simulink model "TRAMI_STEP_AT_vehicle_ver01_Jmaab_R2018b"  (R2018b)
settings: Solver=ode8  StartTime=0  StopTime=end_time  FixedStep=sampling_time  RelTol=1e-3
PreLoadFcn:
  | %init_setting;
values from neighbouring files (symbols this model uses):
  sampling_time = 0.0025    [METI_TRAMI_Thermal_ver01_Jmaab_PreLoad.m]
undefined symbols (not defined in the file or in its folder): ACC_D_Gain, ACC_I_Gain, ACC_P_Gain, ALT_CNT_ALT_OFF_RPM_HYS_rpm, ALT_CNT_ALT_ON_RPM_HYS_rpm, ALT_CNT_Alter_V_BASE_V, ALT_CNT_Alter_V_Kaisei_V, ALT_CNT_flag_disable_kaisei, ALT_CNT_V_Battely_Kudo_V, ALT_PNT_ALT_GDCurrent_A, ALT_PNT_ALT_GDVolt_V, ALT_PNT_Alter_limit_Current_V_table, ALT_PNT_Alter_limit_Current_V_table_x_rpm, ALT_PNT_Alter_trq_Nm_map, ALT_PNT_Alter_trq_Nm_map_x_rpm, ALT_PNT_Alter_trq_Nm_map_y_Current_A, ALT_PNT_Alter_trq_Nm_map_z_Volt_tgt_V, ALT_PNT_eta_pulley_alt, ALT_PNT_Gain_Alt_v_del, ALT_PNT_ratio_pulley_alt, ALT_PNT_Tau_Alternator_V_tgt_s, ALT_PNT_trq_alter_output_LL_Nm, BK_PNT_Pow_UL, BK_PNT_Tau_brake, Brk_LL, Brk_PGain, Brk_UL, BT_PNT_Lo_Capa_lo_batt_F, BT_PNT_Lo_ocv_SOC_lo_batt_OCV_V_table, BT_PNT_Lo_ocv_SOC_lo_batt_OCV_V_table_x_SOC, BT_PNT_Lo_R_lo_batt_ohm, BT_PNT_Lo_SOC_MAX_lo_batt, BT_PNT_Lo_SOC_MIN_lo_batt, BT_PNT_Lo_SOC_START_lo_batt, BT_PNT_Lo_V_start_ocv, DF_PNT_DF_gear, Driver_Brake_Const1, Driver_Brake_Const3, Driver_Brake_Switch_Const2, Driver_Brk_sh, drivmode_ACC, drivmode_CONST, drivmode_GensokuKaisei, drivmode_GensokuRikko, drivmode_STOP, EL_PNT_R_bodyelec_lo_ohm, ENG_CNT_Accel_LL, ENG_CNT_Accel_UL, ENG_CNT_brak_idlestop, ENG_CNT_flag_idle_stop_exe, ENG_CNT_gain_p_per_isc, ENG_CNT_IdleSpeed_Const, ENG_CNT_omg_eng_fuelcut_rpm, ENG_CNT_per_isc_max, ENG_CNT_per_isc_min, ENG_CNT_per_throttle_fuelcut, ENG_CNT_per_throttle_isc_fb, ENG_CNT_Starter_timer_Const_s, ENG_CNT_Throttle_LL, ENG_CNT_Throttle_UL ... (+31)
libraries: METI_Lib_vehicle_model x18, simulink x4, AZAPA_Lib_vehicle_model x1
(part 2 of 3)

== system TRAMI_STEP_AT_vehicle_ver01_Jmaab_R2018b/Vehicle/CNT/TM_CNT ==
  sensor_VL_PNT_BUS : Inport
  sensor_TM_PNT_BUS : Inport  Port=2
  Bus Creator : BusCreator  Inputs=2
  Bus Creator2 : BusCreator  Inputs=12
  Bus Selector1 : BusSelector  OutputSignals=open_accel_per,trq_BK_PNT_Nm,IdleSpeed_Target
  Bus Selector11 : BusSelector  OutputSignals=w_TM_PNT_GearBox_in_radps,w_TM_PNT_GearBox_out_radps,wDiff,T_oil_K,w_TM_PNT_out_radps,trq_FW_PNT_in_unLim_Nm,trq_FW_PNT_in_Nm
  Bus Selector3 : BusSelector  OutputSignals=v_VL_PNT_kmph
  Constant : Constant  Value=500
  Constant1 : Constant  Value=0
  Gain : Gain  Gain=2*pi/60
  Gain1 : Gain  Gain=-1
  Step : Step  Time=5.57  SampleTime=0
  T_PT_TH_K : Subsystem
  Terminator1 : Terminator
  Terminator2 : Terminator
  plant_Connection : Subsystem
  TM_CNT_out : Outport
  tag scope: TM_CNT_CAN_Tx=scoped
  wires:
  Bus Creator/1 -> [TM_CNT_CAN_Tx]  "TM_CNT_CAN_Tx"
  [TM_CNT_CAN_Rx] -> Bus Selector1/1
  Bus Selector1/1 -> plant_Connection/6(accel_position_per)  "<open_accel_per>"
  sensor_VL_PNT_BUS/1 -> Bus Selector3/1
  Bus Selector11/4 -> plant_Connection/4(t_trans_fluid_k)  "<T_oil_K>"
  Bus Selector11/7 -> plant_Connection/13(tau_engine)  "<trq_FW_PNT_in_Nm>"
  Bus Selector11/6 -> plant_Connection/12(tau_engine_target)  "<trq_FW_PNT_in_unLim_Nm>"
  plant_Connection/9(tq_engine_min_req) -> Bus Creator2/9
  plant_Connection/13(flag_lock_up) -> Bus Creator/1, Bus Creator2/11
  plant_Connection/12(gear_ratio) -> Bus Creator/2, Bus Creator2/10
  plant_Connection/7(q_cooler_engine_water) -> Bus Creator2/7
  plant_Connection/6(q_cooler_trans_fluid) -> Bus Creator2/6
  plant_Connection/1(tq_clutch_cap) -> Bus Creator2/1
  plant_Connection/8(tq_engine_max_req) -> Bus Creator2/8
  T_PT_TH_K/1(Out1) -> plant_Connection/5(t_engine_water_k)
  Bus Creator2/1 -> TM_CNT_out/1  "TM_CNT_out"
  Constant/1 -> plant_Connection/15(tau_engine_max_pos)
  plant_Connection/5(i_eop) -> Bus Creator2/5
  plant_Connection/14(lock_up_cap) -> Bus Creator2/12
  Bus Selector11/2 -> plant_Connection/2(w_gearbox_output_radps)  "<w_TM_PNT_GearBox_out_radps>"
  Gain/1 -> plant_Connection/11(w_engine_idle_radps)
  Step/1 -> plant_Connection/7(trans_shifer_position)
  Constant1/1 -> plant_Connection/14(tau_engine_min_pos)
  plant_Connection/3(p_line) -> Bus Creator2/3
  plant_Connection/11(tq_trans_input) -> Terminator2/1
  Bus Selector11/1 -> plant_Connection/1(w_gearbox_input_radps)  "<w_TM_PNT_GearBox_in_radps>"
  plant_Connection/4(i_actuator) -> Bus Creator2/4
  Gain1/1 -> plant_Connection/9(tau_brake)
  sensor_TM_PNT_BUS/1 -> Bus Selector11/1
  plant_Connection/10(r_engine_target) -> Terminator1/1
  Bus Selector11/3 -> plant_Connection/3(w_synchoro_dif_radps)  "<wDiff>"
  plant_Connection/2(f_synchro_n) -> Bus Creator2/2
  Bus Selector11/5 -> plant_Connection/10(w_engine_radps)  "<w_TM_PNT_out_radps>"
  Bus Selector3/1 -> plant_Connection/8(v_vehicle_mps)  "<v_VL_PNT_kmph>"
  Bus Selector1/3 -> Gain/1  "<IdleSpeed_Target>"
  Bus Selector1/2 -> Gain1/1  "<trq_BK_PNT_Nm>"

== system TRAMI_STEP_AT_vehicle_ver01_Jmaab_R2018b/Vehicle/ENG_PNT/ENG_Plant ==
  note: 軸トルクマップ
  note: 燃料消費率マップ
  open_throttle_per : Inport
  flag_fuelcut : Inport  Port=2
  flag_IdleStop : Inport  Port=3
  timing_ignition : Inport  Port=4
  w_ENG_PNT_radps : Inport  Port=5
  Cal_FuelComsunption : Subsystem
  Cal_trq_ENG_jiku : Subsystem
  Gain : Gain  Gain=radpsec2rpm
  Integrator : Integrator
  Model Info : simulink/Model-Wide Utilities/Model Info  Frame=on  DisplayStringWithTags=【注記】 ・エンジンモデルはトルク出力動作させる側が正  HorizontalTextAlignment=Left  LeftAlignmentValue=0.02
  P_cal : METI_Lib_vehicle_model/P_cal  Type_energy=回転運動  Type_output_energy=出力  Power_name=Po_  t_Workspace_Name=ENG_PNT_MECK  P_VariableName=Po_ENG_PNT_MECK  Across_VariableName=w_ENG_PNT_MECK  Throgh_VariableName=tq_ENG_PNT_MECK
  Terminator1 : Terminator
  n_eng_rpm : Outport
  trq_ENG_PNT_Nm : Outport  Port=2
  tag scope: tScope_ENG_speed_rpm=global, tScope_ENG_torq=global, tScope_Fuel=global, tScope_Fuelraio=global
  wires:
  w_ENG_PNT_radps/1 -> Cal_trq_ENG_jiku/5(w_ENG_PNT_radps), P_cal/1, Gain/1, Cal_FuelComsunption/1(w_ENG_PNT_radps)
  Cal_FuelComsunption/1(FuelComsunption) -> [tScope_Fuelraio], Integrator/1
  flag_fuelcut/1 -> Cal_trq_ENG_jiku/2(flag_fuelcut), Cal_FuelComsunption/3(flag_fuelcut)
  flag_IdleStop/1 -> Cal_FuelComsunption/4(flag_IdleStop), Cal_trq_ENG_jiku/3(flag_IdleStop)
  P_cal/1 -> Terminator1/1
  open_throttle_per/1 -> Cal_trq_ENG_jiku/1(open_throttle_per)
  timing_ignition/1 -> Cal_FuelComsunption/5(timing_ignition), Cal_trq_ENG_jiku/4(timing_ignition)
  Integrator/1 -> [tScope_Fuel]
  Gain/1 -> [tScope_ENG_speed_rpm], n_eng_rpm/1  "n_eng_rpm"
  Cal_trq_ENG_jiku/1(trq_ENG_PNT_Nm) -> Cal_FuelComsunption/2(trq_ENG), [tScope_ENG_torq], trq_ENG_PNT_Nm/1, P_cal/2

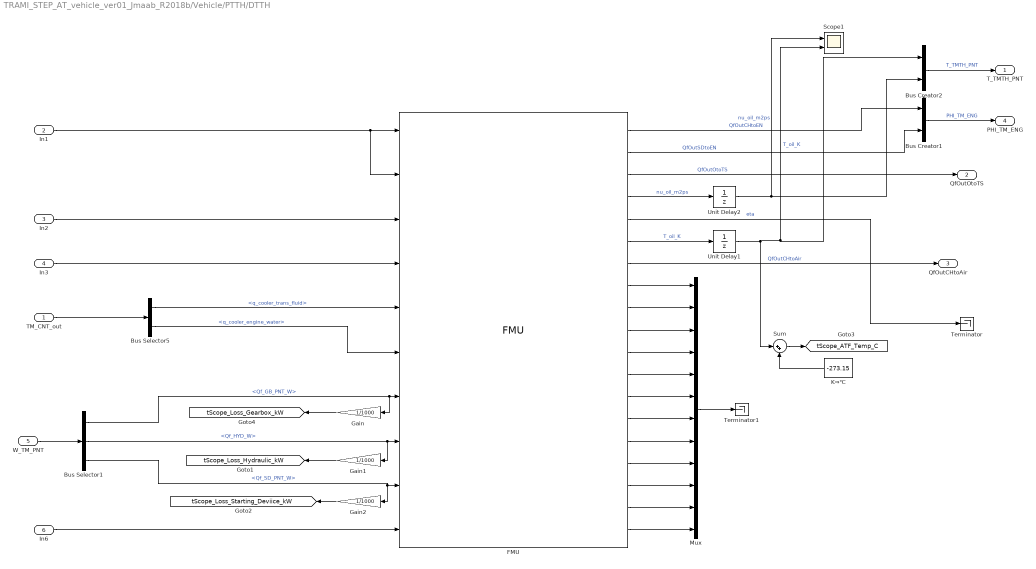
== system TRAMI_STEP_AT_vehicle_ver01_Jmaab_R2018b/Vehicle/PTTH/DTTH ==
  TM_CNT_out : Inport
  In1 : Inport  Port=2
  In2 : Inport  Port=3
  In3 : Inport  Port=4
  W_TM_PNT : Inport  Port=5
  In6 : Inport  Port=6
  Bus Creator1 : BusCreator  Inputs=2
  Bus Creator2 : BusCreator  Inputs=2
  Bus Selector1 : BusSelector  OutputSignals=Qf_GB_PNT_W,Qf_HYD_W,Qf_SD_PNT_W
  Bus Selector5 : BusSelector  OutputSignals=q_cooler_trans_fluid,q_cooler_engine_water
  FMU : FMU  FMUName=ThermalModelAll_CS.fmu  FMUDebugLogging=on  FMUMode=CoSimulation  c1=5000  T0=300  R1=100  T1=300  R2=0.10  R3=100  R4=100  R5=0.006  table1_1_1__1_1_=0.  table1_1_2__1_2_=0.022  table1_2_1__2_1_=10.  table1_2_2__2_2_=0.021  table1_3_1__3_1_=20.  table1_3_2__3_2_=0.021  table1_4_1__4_1_=30.  table1_4_2__4_2_=0.020  table1_5_1__5_1_=40.  table1_5_2__5_2_=0.019  table1_6_1__6_1_=50.  table1_6_2__6_2_=0.018  table1_7_1__7_1_=60.  table1_7_2__7_2_=0.017  table1_8_1__8_1_=70.  table1_8_2__8_2_=0.016  table1_9_1__9_1_=80.  table1_9_2__9_2_=0.015  table1_10_1__10_1_=90.  table1_10_2__10_2_=0.014  table1_11_1__11_1_=100.  table1_11_2__11_2_=0.013  table1_12_1__12_1_=110.  table1_12_2__12_2_=0.012  table1_13_1__13_1_=120.  table1_13_2__13_2_=0.012  table1_14_1__14_1_=130.  table1_14_2__14_2_=0.011  table1_15_1__15_1_=140.  table1_15_2__15_2_=0.011  table1_16_1__16_1_=150.  table1_16_2__16_2_=0.010  table1_17_1__17_1_=160.  table1_17_2__17_2_=0.010  c3=15000  T2=300  fileName1=./DATA/thResistanceOilColler1.txt  tableName1=thResistanceOilColler1  T3=300  c4=10000  R6=0.0007  R7=0.05  Nutable1_1_1__1_1_=-30.  Nutable1_1_2__1_2_=70  Nutable1_2_1__2_1_=0.  Nutable1_2_2__2_2_=70  Nutable1_3_1__3_1_=20.  Nutable1_3_2__3_2_=70  Nutable1_4_1__4_1_=40.  Nutable1_4_2__4_2_=40  Nutable1_5_1__5_1_=60.  Nutable1_5_2__5_2_=23  Nutable1_6_1__6_1_=80.  Nutable1_6_2__6_2_=13  Nutable1_7_1__7_1_=100.  Nutable1_7_2__7_2_=7.5  Nutable1_8_1__8_1_=120.  Nutable1_8_2__8_2_=7.5  EtaTable1_1_1__1_1_=-30.  EtaTable1_1_2__1_2_=70  EtaTable1_2_1__2_1_=0.  EtaTable1_2_2__2_2_=70  EtaTable1_3_1__3_1_=20.  EtaTable1_3_2__3_2_=70  EtaTable1_4_1__4_1_=40.  EtaTable1_4_2__4_2_=40  EtaTable1_5_1__5_1_=60.  EtaTable1_5_2__5_2_=23  EtaTable1_6_1__6_1_=80.  EtaTable1_6_2__6_2_=13  EtaTable1_7_1__7_1_=100.  EtaTable1_7_2__7_2_=7.5  EtaTable1_8_1__8_1_=120.  EtaTable1_8_2__8_2_=7.5  kDammy=1.  c2=30000  settings_dtMin=1e-08  settings_dtMax=0.01  settings_absTol=1e-05  settings_relTol=1e-05  settings_iMode=int32(1)  settings_maxOrder=int32(5)  mask(ThermalModelAll [Co-Simulation, v2.0]){}
      mask Display:
      | disp('ThermalModelAll');
      | port_label('output',1,'QfOutCHtoEN');
      | port_label('output',2,'QfOutSDtoEN');
      | port_label('output',3,'QfOutOCtoTS');
      | port_label('output',4,'nuOil');
      | port_label('output',5,'etaOil');
      | port_label('output',6,'ToutOil');
      | port_label('output',7,'QfOutCHtoAir');
      | port_label('output',8,'ToutOiltoOC');
      | port_label('output',9,'QfOutOCtoOil');
      | port_label('output',10,'ToutSDtoOil');
      | port_label('output',11,'QfOutOiltoSD');
      | port_label('output',12,'ToutSDtoCH');
      | port_label('output',13,'QfOutCHtoSD');
      | port_label('output',14,'ToutOiltoCH');
      | port_label('output',15,'QfoutCHtoOil');
      | port_label('output',16,'QfOiltoGear');
      | port_label('output',17,'ToutGeartoOil');
      | port_label('output',18,'ToutGeartoCH');
      | port_label('output',19,'QfOutCHtoGear');
      | port_label('input',1,'TinENtoCH');
      | port_label('input',2,'TinENtoSD');
      | port_label('input',3,'TinTStoOC');
      | port_label('input',4,'TinAirtoCH');
      | port_label('input',5,'VIdot1OilCooler');
      | port_label('input',6,'VIdot2OilCooler');
      | port_label('input',7,'QfGear');
      | port_label('input',8,'QfOil');
      | port_label('input',9,'QfStartDevice');
      | port_label('input',10,'vCaseHousing');
  Gain : Gain  Gain=1/1000
  Gain1 : Gain  Gain=1/1000
  Gain2 : Gain  Gain=1/1000
  K⇒℃ : Constant  Value=-273.15
  Mux : Mux  Inputs=12
  Scope1 : Scope  NumInputPorts=2
  Sum : Sum  Inputs=|++
  Terminator : Terminator
  Terminator1 : Terminator
  Unit Delay1 : UnitDelay  InitialCondition=8e-5  SampleTime=-1
  Unit Delay2 : UnitDelay  InitialCondition=8e-5  SampleTime=-1
  T_TMTH_PNT : Outport
  QfOutOtoTS : Outport  Port=2
  QfOutCHtoAir : Outport  Port=3
  PHI_TM_ENG : Outport  Port=4
  tag scope: tScope_ATF_Temp_C=global, tScope_Loss_Gearbox_kW=global, tScope_Loss_Hydraulic_kW=global, tScope_Loss_Starting_Deviice_kW=global
  wires:
  FMU/14 -> Mux/7
  Unit Delay2/1 -> Scope1/1, Bus Creator2/2  "nu_oil_m2ps"
  Bus Selector1/1 -> Gain/1, FMU/7  "<Qf_GB_PNT_W>"
  K⇒℃/1 -> Sum/2
  Gain1/1 -> [tScope_Loss_Hydraulic_kW]
  Gain/1 -> [tScope_Loss_Gearbox_kW]
  Unit Delay1/1 -> Bus Creator2/1, Scope1/2, Sum/1  "T_oil_K"
  W_TM_PNT/1 -> Bus Selector1/1
  Gain2/1 -> [tScope_Loss_Starting_Deviice_kW]
  Sum/1 -> [tScope_ATF_Temp_C]
  FMU/18 -> Mux/11
  FMU/16 -> Mux/9
  TM_CNT_out/1 -> Bus Selector5/1
  In1/1 -> FMU/2, FMU/1
  FMU/2 -> Bus Creator1/2  "QfOutSDtoEN"
  FMU/12 -> Mux/5
  FMU/4 -> Unit Delay2/1  "nu_oil_m2ps"
  FMU/17 -> Mux/10
  FMU/8 -> Mux/1
  FMU/19 -> Mux/12
  Bus Selector1/2 -> Gain1/1, FMU/8  "<Qf_HYD_W>"
  FMU/11 -> Mux/4
  FMU/10 -> Mux/3
  FMU/9 -> Mux/2
  Bus Selector1/3 -> Gain2/1, FMU/9  "<Qf_SD_PNT_W>"
  FMU/15 -> Mux/8
  Mux/1 -> Terminator1/1
  FMU/13 -> Mux/6
  FMU/6 -> Unit Delay1/1  "T_oil_K"
  FMU/5 -> Terminator/1  "eta"
  Bus Selector5/2 -> FMU/6  "<q_cooler_engine_water>"
  In6/1 -> FMU/10
  Bus Selector5/1 -> FMU/5  "<q_cooler_trans_fluid>"
  FMU/7 -> QfOutCHtoAir/1  "QfOutCHtoAir"
  FMU/3 -> QfOutOtoTS/1  "QfOutOtoTS"
  In2/1 -> FMU/3
  In3/1 -> FMU/4
  FMU/1 -> Bus Creator1/1  "QfOutCHtoEN"
  Bus Creator2/1 -> T_TMTH_PNT/1  "T_TMTH_PNT"
  Bus Creator1/1 -> PHI_TM_ENG/1  "PHI_TM_ENG"

== system TRAMI_STEP_AT_vehicle_ver01_Jmaab_R2018b/Vehicle/PTTH/ENGTH ==
  PHI_TM_ENG : Inport
  Bus Selector : BusSelector  OutputSignals=QfOutCHtoEN,QfOutSDtoEN
  From Workspace1 : FromWorkspace  VariableName=T_ENG_K  SampleTime=0  OutputAfterFinalValue=Holding final value
  Sum : Sum  Inputs=|++
  Terminator : Terminator
  Terminator1 : Terminator
  ℃⇒K : Constant  Value=273.15
  T_ENG_K : Outport
      settings: AttributesFormatString=|
      | %<Tag>
      | Priority=<%<Priority>>
  wires:
  Bus Selector/2 -> Terminator/1  "<QfOutSDtoEN>"
  From Workspace1/1 -> Sum/1
  ℃⇒K/1 -> Sum/2
  Sum/1 -> T_ENG_K/1  "T_ENG_K"
  PHI_TM_ENG/1 -> Bus Selector/1
  Bus Selector/1 -> Terminator1/1  "<QfOutCHtoEN>"

== system TRAMI_STEP_AT_vehicle_ver01_Jmaab_R2018b/Vehicle/PTTH/PT_TH ==
  Qf_cooler_PT_TH_W : Inport
      settings: AttributesFormatString=|
      | %<Tag>
      | Priority=<%<Priority>>
  From Workspace1 : FromWorkspace  VariableName=T_PT_TH_K  SampleTime=0  OutputAfterFinalValue=Holding final value
  Sum : Sum  Inputs=|++
  Terminator : Terminator
  ℃⇒K : Constant  Value=273.15
  T_PT_TH_K : Outport
      settings: AttributesFormatString=|
      | %<Tag>
      | Priority=<%<Priority>>
  wires:
  Qf_cooler_PT_TH_W/1 -> Terminator/1
  ℃⇒K/1 -> Sum/2
  From Workspace1/1 -> Sum/1
  Sum/1 -> T_PT_TH_K/1  "T_PT_TH_K"

== system TRAMI_STEP_AT_vehicle_ver01_Jmaab_R2018b/Vehicle/PTTH/air ==
  Qf_case_air_W : Inport
      settings: AttributesFormatString=|
      | %<Tag>
      | Priority=<%<Priority>>
  From Workspace1 : FromWorkspace  VariableName=T_air_K  SampleTime=0  OutputAfterFinalValue=Holding final value
  Sum : Sum  Inputs=|++
  Terminator : Terminator
  ℃⇒K : Constant  Value=273.15
  T_air_K : Outport
      settings: AttributesFormatString=|
      | %<Tag>
      | Priority=<%<Priority>>
  wires:
  Qf_case_air_W/1 -> Terminator/1
  From Workspace1/1 -> Sum/1
  ℃⇒K/1 -> Sum/2
  Sum/1 -> T_air_K/1  "T_air_K"

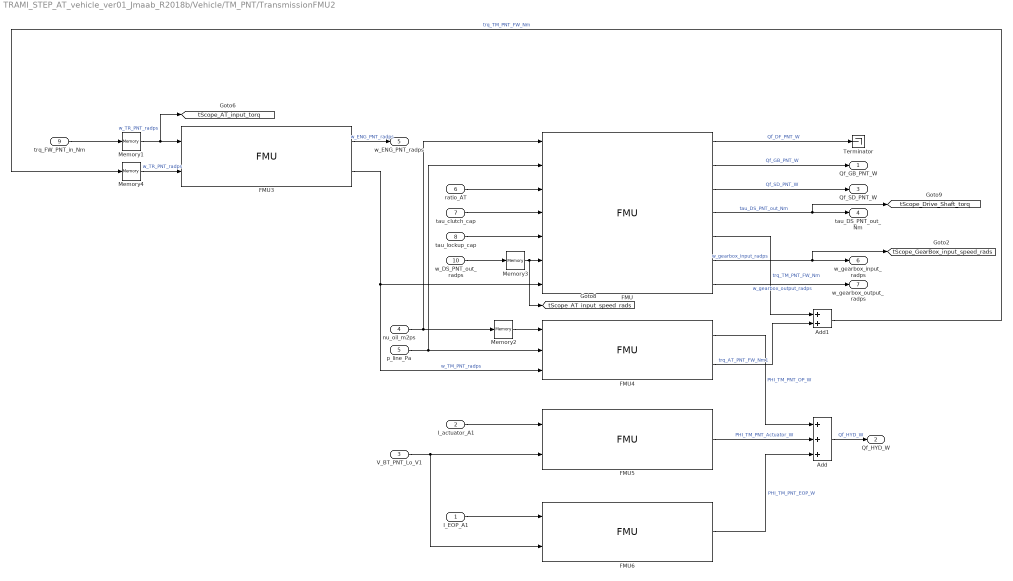
== system TRAMI_STEP_AT_vehicle_ver01_Jmaab_R2018b/Vehicle/TM_PNT/TransmissionFMU2 ==
  I_EOP_A1 : Inport
  I_actuator_A1 : Inport  Port=2
  V_BT_PNT_Lo_V1 : Inport  Port=3
  nu_oil_m2ps : Inport  Port=4
  p_line_Pa : Inport  Port=5
  ratio_AT : Inport  Port=6
  tau_clutch_cap : Inport  Port=7
  tau_lockup_cap : Inport  Port=8
  trq_FW_PNT_in_Nm : Inport  Port=9
  w_DS_PNT_out_radps : Inport  Port=10
  Add : Sum  Inputs=+++
  Add1 : Sum
  FMU : FMU  FMUName=AtDsFmu.fmu  FMUMode=CoSimulation  minsamplestep=2.50000000000000000e-02  binfilename=DISABLED  mask(AtDsFmu [Co-Simulation, v2.0]){}
      mask Display:
      | disp('AtDsFmu');
      | port_label('output',1,'Qf_DF_PNT_W');
      | port_label('output',2,'Qf_GB_PNT_W');
      | port_label('output',3,'Qf_SD_PNT_W');
      | port_label('output',4,'tau_DS_PNT_out_Nm');
      | port_label('output',5,'trq_TM_PNT_FW_Nm');
      | port_label('output',6,'w_gearbox_input_radps');
      | port_label('output',7,'w_gearbox_output_radps');
      | port_label('input',1,'nu_oil_m2ps');
      | port_label('input',2,'p_line_Pa');
      | port_label('input',3,'ratio_AT');
      | port_label('input',4,'tau_clutch_cap');
      | port_label('input',5,'tau_lockup_cap');
      | port_label('input',6,'w_DS_PNT_out_radps');
      | port_label('input',7,'w_TM_PNT_FW_radps');
  FMU3 : FMU  FMUName=Flywheel.fmu  FMUMode=CoSimulation  Iwh=4.00000000000000000e-01  minsamplestep=2.50000000000000000e-02  binfilename=DISABLED  mask(Flywheel [Co-Simulation, v2.0]){}
      mask Display:
      | disp('Flywheel');
      | port_label('output',1,'w_ENG_PNT_radps');
      | port_label('output',2,'w_TM_PNT_FW_radps');
      | port_label('input',1,'trq_ENG_PNT_in_Nm');
      | port_label('input',2,'trq_TM_PNT_FW_Nm');
  FMU4 : FMU  FMUName=OilPump.fmu  FMUMode=CoSimulation  Oil_Viscosity_Breakpoint_2=1.02000000000000000e-05  Oil_Viscosity_Breakpoint_3=1.69000000000000000e-05  Oil_Viscosity_Breakpoint_4=3.12000000000000000e-05  minsamplestep=2.50000000000000000e-02  binfilename=DISABLED  mask(OilPump [Co-Simulation, v2.0]){}
      mask Display:
      | disp('OilPump');
      | port_label('output',1,'PHI_TM_PNT_OP_W');
      | port_label('output',2,'trq_AT_PNT_Nm1');
      | port_label('input',1,'nu_oil_m2ps');
      | port_label('input',2,'p_Line_Pa');
      | port_label('input',3,'w_AT_PNT_radps1');
  FMU5 : FMU  FMUName=ActuatorELoss.fmu  FMUMode=CoSimulation  minsamplestep=2.50000000000000000e-02  binfilename=DISABLED  mask(ActuatorELoss [Co-Simulation, v2.0]){}
      mask Display:
      | disp('ActuatorELoss');
      | port_label('output',1,'PHI_TM_PNT_Actuator_W');
      | port_label('input',1,'I_actuator_A');
      | port_label('input',2,'V_BT_PNT_Lo_V');
  FMU6 : FMU  FMUName=EOPELoss.fmu  FMUMode=CoSimulation  minsamplestep=2.50000000000000000e-02  binfilename=DISABLED  mask(EOPELoss [Co-Simulation, v2.0]){}
      mask Display:
      | disp('EOPELoss');
      | port_label('output',1,'PHI_TM_PNT_EOP_W');
      | port_label('input',1,'I_EOP_A');
      | port_label('input',2,'V_BT_PNT_Lo_V');
  Memory{1..4} (4 alike) : Memory
  Terminator : Terminator
  Qf_GB_PNT_W : Outport
  Qf_HYD_W : Outport  Port=2
  Qf_SD_PNT_W : Outport  Port=3
  tau_DS_PNT_out_Nm : Outport  Port=4
  w_ENG_PNT_radps : Outport  Port=5
  w_gearbox_input_radps : Outport  Port=6
  w_gearbox_output_radps : Outport  Port=7
  tag scope: tScope_AT_input_speed_rads=global, tScope_AT_input_torq=global, tScope_Drive_Shaft_torq=global, tScope_GearBox_input_speed_rads=global
  wires:
  FMU3/1 -> w_ENG_PNT_radps/1  "w_ENG_PNT_radps"
  FMU5/1 -> Add/2  "PHI_TM_PNT_Actuator_W"
  FMU6/1 -> Add/3  "PHI_TM_PNT_EOP_W"
  FMU4/1 -> Add/1  "PHI_TM_PNT_OP_W"
  Add/1 -> Qf_HYD_W/1  "Qf_HYD_W"
  FMU4/2 -> Add1/2  "trq_AT_PNT_FW_Nm1"
  I_EOP_A1/1 -> FMU6/1
  I_actuator_A1/1 -> FMU5/1
  V_BT_PNT_Lo_V1/1 -> FMU6/2, FMU5/2
  trq_FW_PNT_in_Nm/1 -> Memory1/1
  p_line_Pa/1 -> FMU/2, FMU4/2
  nu_oil_m2ps/1 -> FMU/1, Memory2/1
  FMU3/2 -> FMU/7, FMU4/3  "w_TM_PNT_radps"
  Add1/1 -> Memory4/1  "trq_TM_PNT_FW_Nm"
  ratio_AT/1 -> FMU/3
  tau_clutch_cap/1 -> FMU/4
  tau_lockup_cap/1 -> FMU/5
  FMU/5 -> Add1/1  "trq_TM_PNT_FW_Nm"
  FMU/1 -> Terminator/1  "Qf_DF_PNT_W"
  FMU/2 -> Qf_GB_PNT_W/1  "Qf_GB_PNT_W"
  FMU/3 -> Qf_SD_PNT_W/1  "Qf_SD_PNT_W"
  FMU/4 -> [tScope_Drive_Shaft_torq], tau_DS_PNT_out_Nm/1  "tau_DS_PNT_out_Nm"
  FMU/6 -> [tScope_GearBox_input_speed_rads], w_gearbox_input_radps/1  "w_gearbox_input_radps"
  FMU/7 -> w_gearbox_output_radps/1  "w_gearbox_output_radps"
  Memory2/1 -> FMU4/1
  Memory1/1 -> [tScope_AT_input_torq], FMU3/1  "w_TR_PNT_radps"
  w_DS_PNT_out_radps/1 -> Memory3/1
  Memory4/1 -> FMU3/2  "w_TR_PNT_radps"
  Memory3/1 -> [tScope_AT_input_speed_rads], FMU/6

== system TRAMI_STEP_AT_vehicle_ver01_Jmaab_R2018b/Driver/Caliculate_Opeining_Accel/FB/Filter ==
  In1 : Inport
  Gain3 : Gain  Gain=10
  Gain4 : Gain  Gain=0.1
  Rounding Function : Rounding  Operator=round
  Out1 : Outport
  wires:
  Rounding Function/1 -> Gain4/1
  In1/1 -> Gain3/1
  Gain3/1 -> Rounding Function/1
  Gain4/1 -> Out1/1

== system TRAMI_STEP_AT_vehicle_ver01_Jmaab_R2018b/Driver/Caliculate_Opeining_Accel/FF/Air_Resistance ==
  V_tgt : Inport
  V_wind : Constant  Value=VL_PNT_V_wind
  cal_Air_resi1 : METI_Lib_vehicle_model/vehicle_model/cal_Air_resi  Vel_max=200
  F_air_resi : Outport
  wires:
  V_tgt/1 -> cal_Air_resi1/1
  V_wind/1 -> cal_Air_resi1/2
  cal_Air_resi1/1 -> F_air_resi/1

== system TRAMI_STEP_AT_vehicle_ver01_Jmaab_R2018b/Driver/Caliculate_Opeining_Accel/FF/Cal_M_ENG_jiku2 ==
  note: 軸トルクマップ
  FF_trq_accel_Nm : Inport
  pre_n_eng_rpm : Inport  Port=2
  2-D Lookup Table : Lookup_n-D  BreakpointsForDimension1=ENG_trq_rev  BreakpointsForDimension2=ENG_rpm  Table=ENG_throttle_rev  ExtrapMethod=Clip  UseLastTableValue=on  RndMeth=Simplest  InputSameDT=on
  2-D Lookup Table1 : Lookup_n-D  BreakpointsForDimension1=ENG_PNT_trq_Nm_map_y_throttle  BreakpointsForDimension2=ENG_PNT_trq_Nm_map_x_rpm  Table=ENG_PNT_trq_Nm_map  ExtrapMethod=Clip  UseLastTableValue=on  RndMeth=Simplest  InputSameDT=on
  Constant : Constant  Value=0
  Subsystem : Subsystem
  Sum : Sum  Inputs=|++
  FF_open_accel_per : Outport
  wires:
  FF_trq_accel_Nm/1 -> Sum/1
  2-D Lookup Table/1 -> Subsystem/1(In1)
  pre_n_eng_rpm/1 -> 2-D Lookup Table/2, 2-D Lookup Table1/2
  Constant/1 -> 2-D Lookup Table1/1
  Sum/1 -> 2-D Lookup Table/1
  2-D Lookup Table1/1 -> Sum/2
  Subsystem/1(Out1) -> FF_open_accel_per/1

== system TRAMI_STEP_AT_vehicle_ver01_Jmaab_R2018b/Driver/Caliculate_Opeining_Accel/FF/Inertial_Resistance ==
  V_tgt : Inport
  Constant : Constant  Value=M
  Derivative : Derivative
  Divide : Product  OutDataTypeStr=Inherit: Same as first input
  F_Inertia : Outport
  wires:
  Constant/1 -> Divide/2
  Derivative/1 -> Divide/1
  Divide/1 -> F_Inertia/1
  V_tgt/1 -> Derivative/1

== system TRAMI_STEP_AT_vehicle_ver01_Jmaab_R2018b/Driver/Caliculate_Opeining_Accel/FF/Rolling_Resistance ==
  note: 20151211修正
      |
      | 空気抵抗と表現を統一する、ため
      | -1のGainを削除
  V_tgt : Inport
  cal_roll_resi1 : METI_Lib_vehicle_model/vehicle_model/cal_roll_resi  Myu_tire=myu  Vehicle_Mass=M  Gravi_acc=g
  F_rollresi : Outport
  wires:
  V_tgt/1 -> cal_roll_resi1/1
  cal_roll_resi1/1 -> F_rollresi/1

== system TRAMI_STEP_AT_vehicle_ver01_Jmaab_R2018b/Vehicle/ALT_PNT/Subsystem/I_alt_cal ==
  target_volt_ALT_V : Inport
  volt_BT_PNT_Lo_V : Inport  Port=2
  rpm_alt : Inport  Port=3
  Add : Sum
  Cal_I_alt_P_control : Subsystem
  Cal_I_alt_base : Subsystem
  Constant : Constant  Value=12
  Constant4 : Constant  Value=0
  Limit_Current_Max : Lookup_n-D  NumberOfTableDimensions=1  BreakpointsForDimension1=ALT_PNT_Alter_limit_Current_V_table_x_rpm  Table=ALT_PNT_Alter_limit_Current_V_table  ExtrapMethod=Clip  UseLastTableValue=on  RndMeth=Simplest  InputSameDT=on
  MinMax2 : MinMax  Function=max  Inputs=2
  Sum1 : Sum  Inputs=|+-
  Sum2 : Sum  Inputs=-+|
  電圧比較 : MinMax  Inputs=2
  I_alt : Outport
  wires:
  target_volt_ALT_V/1 -> Sum1/1, Sum2/2
  volt_BT_PNT_Lo_V/1 -> Sum2/1
  rpm_alt/1 -> Limit_Current_Max/1
  Constant4/1 -> MinMax2/2
  Limit_Current_Max/1 -> MinMax2/1  "I_limit_ALT"
  電圧比較/1 -> I_alt/1
  Add/1 -> 電圧比較/2
  Sum2/1 -> Cal_I_alt_P_control/1(V_delt_tgt)
  MinMax2/1 -> 電圧比較/1
  Constant/1 -> Sum1/2
  Sum1/1 -> Cal_I_alt_base/1(V_delt_tgt)
  Cal_I_alt_P_control/1(I_alt_base) -> Add/1
  Cal_I_alt_base/1(I_alt_base) -> Add/2

== system TRAMI_STEP_AT_vehicle_ver01_Jmaab_R2018b/Vehicle/ALT_PNT/Subsystem/Torque_Guard ==
  current_ALT_PNT_A : Inport
  V_ALT_PNT : Inport  Port=2
  n_ROT_slavepulley12_rpm : Inport  Port=3
  ALT_GDCurrent : Inport  Port=4
  ALT_GDVolt : Inport  Port=5
  Caliculate_Axes_Torque1 : Lookup_n-D  NumberOfTableDimensions=3  BreakpointsForDimension1=ALT_PNT_Alter_trq_Nm_map_x_rpm  BreakpointsForDimension2=ALT_PNT_Alter_trq_Nm_map_y_Current_A  BreakpointsForDimension3=ALT_PNT_Alter_trq_Nm_map_z_Volt_tgt_V  Table=ALT_PNT_Alter_trq_Nm_map  RndMeth=Simplest  InputSameDT=on
  Caliculate_Axes_Torque2 : Lookup_n-D  NumberOfTableDimensions=3  BreakpointsForDimension1=ALT_PNT_Alter_trq_Nm_map_x_rpm  BreakpointsForDimension2=ALT_PNT_Alter_trq_Nm_map_y_Current_A  BreakpointsForDimension3=ALT_PNT_Alter_trq_Nm_map_z_Volt_tgt_V  Table=ALT_PNT_Alter_trq_Nm_map  RndMeth=Simplest  InputSameDT=on
  Constant3 : Constant  Value=ALT_PNT_trq_alter_output_LL_Nm
  MinMax : MinMax  Inputs=2
  MinMax1 : MinMax  Function=max  Inputs=2
  trq_trqsource : Outport
  wires:
  ALT_GDCurrent/1 -> Caliculate_Axes_Torque2/2
  Caliculate_Axes_Torque2/1 -> MinMax/2
  MinMax/1 -> MinMax1/1
  Caliculate_Axes_Torque1/1 -> MinMax/1
  Constant3/1 -> MinMax1/2
  ALT_GDVolt/1 -> Caliculate_Axes_Torque2/3
  MinMax1/1 -> trq_trqsource/1
  V_ALT_PNT/1 -> Caliculate_Axes_Torque1/3
  current_ALT_PNT_A/1 -> Caliculate_Axes_Torque1/2
  n_ROT_slavepulley12_rpm/1 -> Caliculate_Axes_Torque2/1, Caliculate_Axes_Torque1/1

== system TRAMI_STEP_AT_vehicle_ver01_Jmaab_R2018b/Vehicle/BT_PNT_Lo/Cal_SOC/Subsystem4 ==
  In1 : Inport
  In2 : Inport  Port=2
  To Workspace : ToWorkspace  VariableName=SOC_LoBat  SampleTime=-1
      settings: Decimation=num_tws_mabiki
  To Workspace1 : ToWorkspace  VariableName=Asec_LoBat  SampleTime=-1
      settings: Decimation=num_tws_mabiki
  wires:
  In1/1 -> To Workspace/1
  In2/1 -> To Workspace1/1

== system TRAMI_STEP_AT_vehicle_ver01_Jmaab_R2018b/Vehicle/CNT/ALT_CNT/ALT_Ctrl ==
  note: 【発電禁止条件】
      | 下記条件いずれかが成立時はオルタネータの発電を禁止する
      |   (2)エンジン停止中
      |   (3)エンジン始動中(下記エンジン回転数で判定)
      |      ene ≦ ALT_ON_RPM_HYS(1000[rpm])
      |                    ヒスあり(400[rpm])
  note: 【強制回生モード切替条件】
  note: 【回生モード切替条件】
      | 減速時FC中
  note: 例) 12[V]
  note: 例) 14[V]
  note: 例) 13.5[V]
  SOC_BT_PNT_Lo_PCT : Inport
  flag_fuelcut : Inport  Port=2
  flag_IdleStop : Inport  Port=3
  n_eng_rpm : Inport  Port=4
  Constant : Constant  Value=ALT_CNT_Alter_V_Kaisei_V
  Constant1 : Constant  Value=ALT_CNT_V_Battely_Kudo_V
  Constant2 : Constant  Value=ALT_CNT_flag_disable_kaisei
  Constant3 : Constant  Value=ALT_CNT_Alter_V_BASE_V
  Constant4 : Constant  Value=BT_PNT_Lo_SOC_MAX_lo_batt
  Logical Operator : Logic  Operator=OR  Inputs=3  AllPortsSameDT=off  OutDataTypeStr=boolean
  Logical Operator1 : Logic  AllPortsSameDT=off  OutDataTypeStr=boolean
  Logical Operator2 : Logic  Operator=NOT  AllPortsSameDT=off  OutDataTypeStr=boolean
  Relational Operator : RelationalOperator  OutDataTypeStr=boolean  RndMeth=Nearest
  Relay1 : Relay  OnSwitchValue=ALT_CNT_ALT_ON_RPM_HYS_rpm  OffSwitchValue=ALT_CNT_ALT_OFF_RPM_HYS_rpm  OnOutputValue=0  OffOutputValue=1
  Switch1 : Switch  Criteria=u2 > Threshold  Threshold=0.5
  Switch3 : Switch  Criteria=u2 > Threshold  Threshold=0.5
  target_volt_ALT_V : Outport
  wires:
  Switch3/1 -> target_volt_ALT_V/1  "target_volt_ALT_V"
  Constant3/1 -> Switch3/1
  Logical Operator2/1 -> Logical Operator1/2
  SOC_BT_PNT_Lo_PCT/1 -> Relational Operator/1
  Constant2/1 -> Switch3/2
  flag_fuelcut/1 -> Logical Operator1/1
  Relational Operator/1 -> Logical Operator/3
  Constant4/1 -> Relational Operator/2
  Logical Operator1/1 -> Switch1/2
  Logical Operator/1 -> Logical Operator2/1
  Constant/1 -> Switch1/1
  Relay1/1 -> Logical Operator/2
  Switch1/1 -> Switch3/3
  Constant1/1 -> Switch1/3
  flag_IdleStop/1 -> Logical Operator/1
  n_eng_rpm/1 -> Relay1/1

== system TRAMI_STEP_AT_vehicle_ver01_Jmaab_R2018b/Vehicle/CNT/BK_CNT/BK_Ctrl ==
  open_brake_per_in : Inport
  trq_BK_PNT_Nm_in : Inport  Port=2
  open_brake_per : Outport
  trq_BK_PNT_Nm : Outport  Port=2
  wires:
  open_brake_per_in/1 -> open_brake_per/1
  trq_BK_PNT_Nm_in/1 -> trq_BK_PNT_Nm/1

== system TRAMI_STEP_AT_vehicle_ver01_Jmaab_R2018b/Vehicle/CNT/CAN/ALT_CNT ==
  note: ALT_Ctrl
  Pwtr_CAN : Inport
  Bus Creator2 : BusCreator  Inputs=3
  Bus Selector3 : BusSelector  OutputSignals=ENG_CNT_CAN_Tx
  Bus Selector4 : BusSelector  OutputSignals=flag_fuelcut,flag_IdleStop,n_eng_rpm
  tag scope: ALT_CNT_CAN_Rx=scoped
  wires:
  Bus Selector4/2 -> Bus Creator2/2  "<flag_IdleStop>"
  Bus Selector4/3 -> Bus Creator2/3  "<n_eng_rpm>"
  Pwtr_CAN/1 -> Bus Selector3/1
  Bus Creator2/1 -> [ALT_CNT_CAN_Rx]  "ALT_CNT_CAN_Rx"
  Bus Selector4/1 -> Bus Creator2/1  "<flag_fuelcut>"
  Bus Selector3/1 -> Bus Selector4/1  "<ENG_CNT_CAN_Tx>"

== system TRAMI_STEP_AT_vehicle_ver01_Jmaab_R2018b/Vehicle/CNT/CAN/BK_CNT ==
  note: ENG_Ctrl
  Pwtr_CAN : Inport
  Bus Selector1 : BusSelector  OutputSignals=TM_CNT_CAN_Tx
  Bus Selector2 : BusSelector  OutputSignals=flag_lock_up
  Terminator : Terminator
  BK_CNT_CAN_Tx : Outport
  wires:
  [BK_CNT_CAN_Tx] -> BK_CNT_CAN_Tx/1
  Pwtr_CAN/1 -> Bus Selector1/1
  Bus Selector2/1 -> Terminator/1  "<flag_lock_up>"
  Bus Selector1/1 -> Bus Selector2/1  "<TM_CNT_CAN_Tx>"

== system TRAMI_STEP_AT_vehicle_ver01_Jmaab_R2018b/Vehicle/CNT/CAN/ENG_CNT ==
  note: ENG_Ctrl
  Pwtr_CAN : Inport
  Bus Creator3 : BusCreator  Inputs=1
  Bus Selector1 : BusSelector  OutputSignals=TM_CNT_CAN_Tx
  Bus Selector2 : BusSelector  OutputSignals=flag_lock_up
  ENG_CNT_CAN_Tx : Outport
  tag scope: ENG_CNT_CAN_Rx=scoped
  wires:
  Bus Creator3/1 -> [ENG_CNT_CAN_Rx]  "ENG_CNT_CAN_Rx"
  Bus Selector1/1 -> Bus Selector2/1  "<TM_CNT_CAN_Tx>"
  Bus Selector2/1 -> Bus Creator3/1  "<flag_lock_up>"
  Pwtr_CAN/1 -> Bus Selector1/1
  [ENG_CNT_CAN_Tx] -> ENG_CNT_CAN_Tx/1

== system TRAMI_STEP_AT_vehicle_ver01_Jmaab_R2018b/Vehicle/CNT/CAN/Pwtr_CAN ==
  note: 通信遅れ無し
  ENG_CNT_CAN_Tx : Inport
  TM_CNT_CAN_Tx : Inport  Port=2
  BK_CNT_CAN_Tx : Inport  Port=3
  Bus Creator8 : BusCreator  Inputs=3
  Pwtr_CAN : Outport
  wires:
  ENG_CNT_CAN_Tx/1 -> Bus Creator8/1
  TM_CNT_CAN_Tx/1 -> Bus Creator8/2
  Bus Creator8/1 -> Pwtr_CAN/1  "Pwtr_CAN"
  BK_CNT_CAN_Tx/1 -> Bus Creator8/3

== system TRAMI_STEP_AT_vehicle_ver01_Jmaab_R2018b/Vehicle/CNT/CAN/TM_CNT ==
  note: TM_Ctrl
  Pwtr_CAN : Inport
  Bus Creator4 : BusCreator  Inputs=3
  Bus Selector1 : BusSelector  OutputSignals=BK_CNT_CAN_Tx
  Bus Selector2 : BusSelector  OutputSignals=trq_BK_PNT_Nm
  Bus Selector5 : BusSelector  OutputSignals=ENG_CNT_CAN_Tx
  Bus Selector6 : BusSelector  OutputSignals=open_accel_per,IdleSpeed_Target
  TM_CNT_CAN_Tx : Outport
  tag scope: TM_CNT_CAN_Rx=scoped
  wires:
  Bus Selector5/1 -> Bus Selector6/1  "<ENG_CNT_CAN_Tx>"
  Bus Selector6/1 -> Bus Creator4/1  "<open_accel_per>"
  Pwtr_CAN/1 -> Bus Selector1/1, Bus Selector5/1
  Bus Creator4/1 -> [TM_CNT_CAN_Rx]  "TM_CNT_CAN_Rx"
  [TM_CNT_CAN_Tx] -> TM_CNT_CAN_Tx/1
  Bus Selector6/2 -> Bus Creator4/2  "<IdleSpeed_Target>"
  Bus Selector1/1 -> Bus Selector2/1  "<BK_CNT_CAN_Tx>"
  Bus Selector2/1 -> Bus Creator4/3  "<trq_BK_PNT_Nm>"

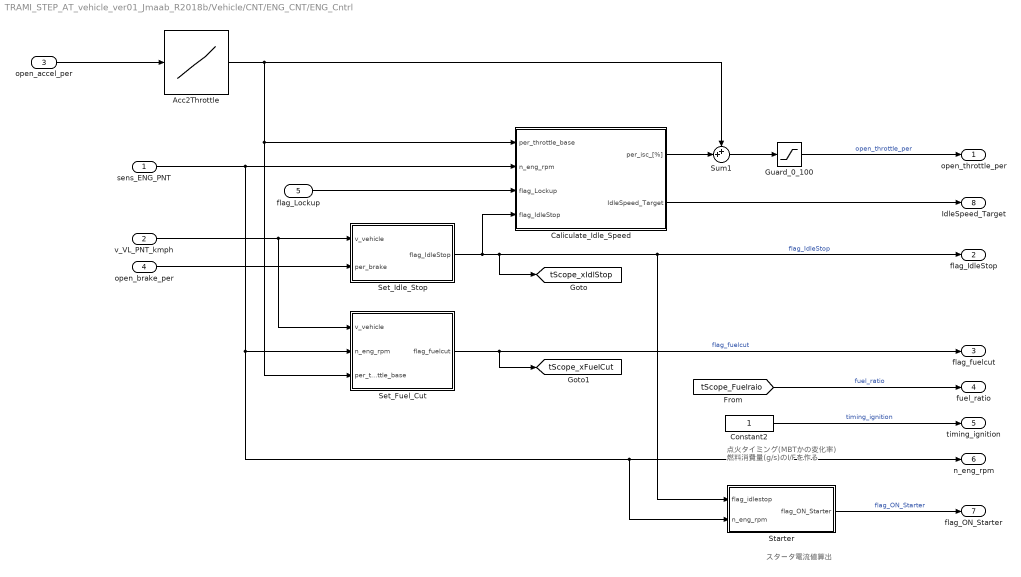
== system TRAMI_STEP_AT_vehicle_ver01_Jmaab_R2018b/Vehicle/CNT/ENG_CNT/ENG_Cntrl ==
  note: 点火タイミング(MBTかの変化率)
      | 燃料消費量(g/s)のI/Fを作る
  note: スタータ電流値算出
  sens_ENG_PNT : Inport
  v_VL_PNT_kmph : Inport  Port=2
  open_accel_per : Inport  Port=3
  open_brake_per : Inport  Port=4
  flag_Lockup : Inport  Port=5
  Acc2Throttle : Lookup_n-D  NumberOfTableDimensions=1  BreakpointsForDimension1=[ENG_CNT_Accel_LL:ENG_CNT_Accel_UL]  Table=[ENG_CNT_Throttle_LL:ENG_CNT_Throttle_UL]  RndMeth=Simplest  InputSameDT=on
  Caliculate_Idle_Speed : Subsystem
  Constant2 : Constant
  Guard_0_100 : Saturate  UpperLimit=ENG_CNT_Throttle_UL  LowerLimit=ENG_CNT_Throttle_LL
  Set_Fuel_Cut : Subsystem
  Set_Idle_Stop : Subsystem
  Starter : Subsystem
  Sum1 : Sum  Inputs=++|
  open_throttle_per : Outport
  flag_IdleStop : Outport  Port=2
  flag_fuelcut : Outport  Port=3
  fuel_ratio : Outport  Port=4
  timing_ignition : Outport  Port=5
  n_eng_rpm : Outport  Port=6
  flag_ON_Starter : Outport  Port=7
  IdleSpeed_Target : Outport  Port=8
  tag scope: tScope_xFuelCut=global, tScope_xIdlStop=global
  wires:
  Set_Idle_Stop/1(flag_IdleStop) -> Caliculate_Idle_Speed/4(flag_IdleStop), flag_IdleStop/1, Starter/1(flag_idlestop), [tScope_xIdlStop]  "flag_IdleStop"
  Constant2/1 -> timing_ignition/1  "timing_ignition"
  sens_ENG_PNT/1 -> Caliculate_Idle_Speed/2(n_eng_rpm), Set_Fuel_Cut/2(n_eng_rpm), n_eng_rpm/1, Starter/2(n_eng_rpm)
  Sum1/1 -> Guard_0_100/1
  Set_Fuel_Cut/1(flag_fuelcut) -> flag_fuelcut/1, [tScope_xFuelCut]  "flag_fuelcut"
  open_accel_per/1 -> Acc2Throttle/1
  Acc2Throttle/1 -> Sum1/1, Caliculate_Idle_Speed/1(per_throttle_base), Set_Fuel_Cut/3(per_throttle_base)
  Starter/1(flag_ON_Starter) -> flag_ON_Starter/1  "flag_ON_Starter"
  open_brake_per/1 -> Set_Idle_Stop/2(per_brake)
  [tScope_Fuelraio] -> fuel_ratio/1  "fuel_ratio"
  v_VL_PNT_kmph/1 -> Set_Idle_Stop/1(v_vehicle), Set_Fuel_Cut/1(v_vehicle)
  Caliculate_Idle_Speed/1(per_isc_[%]) -> Sum1/2
  Guard_0_100/1 -> open_throttle_per/1  "open_throttle_per"
  flag_Lockup/1 -> Caliculate_Idle_Speed/3(flag_Lockup)
  Caliculate_Idle_Speed/2(IdleSpeed_Target) -> IdleSpeed_Target/1

== system TRAMI_STEP_AT_vehicle_ver01_Jmaab_R2018b/Vehicle/CNT/TM_CNT/T_PT_TH_K ==
  From Workspace1 : FromWorkspace  VariableName=T_PT_TH_K  SampleTime=0  OutputAfterFinalValue=Holding final value
  Sum2 : Sum  Inputs=|++
  ℃⇒K : Constant  Value=273.15
  Out1 : Outport
  wires:
  From Workspace1/1 -> Sum2/1
  ℃⇒K/1 -> Sum2/2
  Sum2/1 -> Out1/1

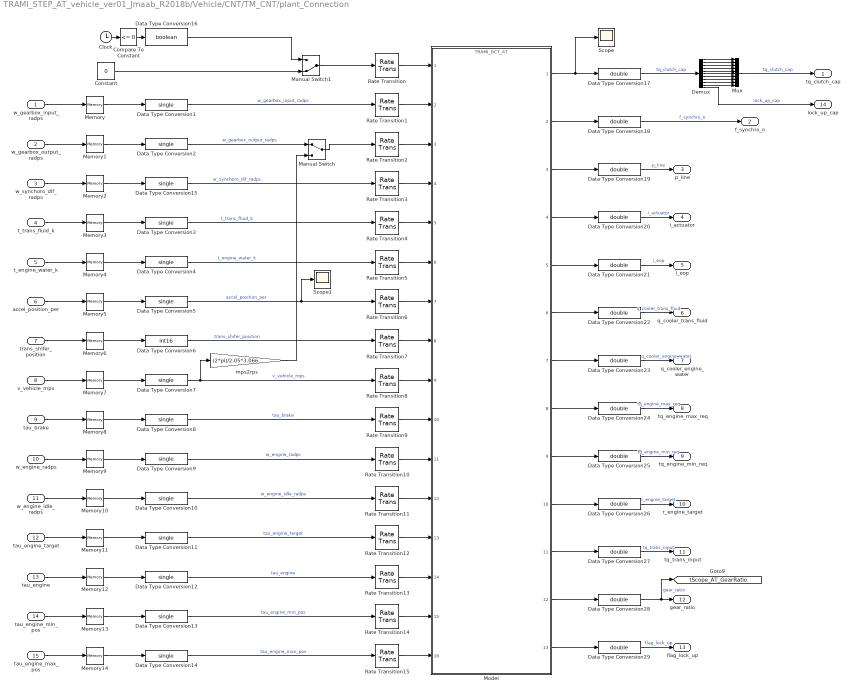
== system TRAMI_STEP_AT_vehicle_ver01_Jmaab_R2018b/Vehicle/CNT/TM_CNT/plant_Connection ==
  w_gearbox_input_radps : Inport
  w_gearbox_output_radps : Inport  Port=2
  w_synchoro_dif_radps : Inport  Port=3
  t_trans_fluid_k : Inport  Port=4
  t_engine_water_k : Inport  Port=5
  accel_position_per : Inport  Port=6
  trans_shifer_position : Inport  Port=7
  v_vehicle_mps : Inport  Port=8
  tau_brake : Inport  Port=9
  w_engine_radps : Inport  Port=10
  w_engine_idle_radps : Inport  Port=11
  tau_engine_target : Inport  Port=12
  tau_engine : Inport  Port=13
  tau_engine_min_pos : Inport  Port=14
  tau_engine_max_pos : Inport  Port=15
  Clock : Clock
  Compare To Constant : simulink/Logic and Bit Operations/Compare To Constant  relop=<=  const=0  OutDataTypeStr=boolean
  Constant : Constant  Value=0  OutDataTypeStr=boolean
  Data Type Conversion{1..5,7..15} (14 alike) : DataTypeConversion  OutDataTypeStr=single
  Data Type Conversion16 : DataTypeConversion  OutDataTypeStr=boolean
  Data Type Conversion{17..29} (13 alike) : DataTypeConversion  OutDataTypeStr=double
  Data Type Conversion6 : DataTypeConversion  OutDataTypeStr=int16
  Demux : Demux  Outputs=11
  Manual Switch : ManualSwitch
  Manual Switch1 : ManualSwitch  CurrentSetting=0
  Memory{,1..14} (15 alike) : Memory
  Model : ModelReference  ModelNameDialog=TRAMI_DCT_AT.slx  SimulationMode=Normal  ModelReferenceVersion=1.20
  Mux : Mux  Inputs=10
  Rate Transition{,1..15} (16 alike) : RateTransition
  Scope : Scope
  Scope1 : Scope
  mps2rps : Gain  Gain=(2*pi)/2.05*3.066
  tq_clutch_cap : Outport
  f_synchro_n : Outport  Port=2
  p_line : Outport  Port=3
  i_actuator : Outport  Port=4
  i_eop : Outport  Port=5
  q_cooler_trans_fluid : Outport  Port=6
  q_cooler_engine_water : Outport  Port=7
  tq_engine_max_req : Outport  Port=8
  tq_engine_min_req : Outport  Port=9
  r_engine_target : Outport  Port=10
  tq_trans_input : Outport  Port=11
  gear_ratio : Outport  Port=12
  flag_lock_up : Outport  Port=13
  lock_up_cap : Outport  Port=14
  tag scope: tScope_AT_GearRatio=global
  wires:
  Manual Switch1/1 -> Rate Transition/1
  Compare To Constant/1 -> Data Type Conversion16/1
  Clock/1 -> Compare To Constant/1
  Data Type Conversion16/1 -> Manual Switch1/1
  Manual Switch/1 -> Rate Transition2/1
  accel_position_per/1 -> Memory5/1
  Model/10 -> Data Type Conversion26/1
  tau_engine_min_pos/1 -> Memory13/1
  tau_engine/1 -> Memory12/1
  Model/2 -> Data Type Conversion18/1
  w_synchoro_dif_radps/1 -> Memory2/1
  t_trans_fluid_k/1 -> Memory3/1
  Model/4 -> Data Type Conversion20/1
  Model/3 -> Data Type Conversion19/1
  Model/1 -> Scope/1, Data Type Conversion17/1
  Model/11 -> Data Type Conversion27/1
  tau_engine_target/1 -> Memory11/1
  mps2rps/1 -> Manual Switch/2
  v_vehicle_mps/1 -> Memory7/1
  Model/5 -> Data Type Conversion21/1
  Data Type Conversion8/1 -> Rate Transition9/1  "tau_brake"
  trans_shifer_position/1 -> Memory6/1
  Data Type Conversion5/1 -> Rate Transition6/1, Scope1/1  "accel_position_per"
  Model/9 -> Data Type Conversion25/1
  w_gearbox_input_radps/1 -> Memory/1
  Data Type Conversion2/1 -> Manual Switch/1  "w_gearbox_output_radps"
  Data Type Conversion1/1 -> Rate Transition1/1  "w_gearbox_input_radps"
  Data Type Conversion9/1 -> Rate Transition10/1  "w_engine_radps"
  Model/6 -> Data Type Conversion22/1
  w_engine_idle_radps/1 -> Memory10/1
  Data Type Conversion15/1 -> Rate Transition3/1  "w_synchoro_dif_radps"
  Model/13 -> Data Type Conversion29/1
  Data Type Conversion13/1 -> Rate Transition14/1  "tau_engine_min_pos"
  Data Type Conversion14/1 -> Rate Transition15/1  "tau_engine_max_pos"
  Data Type Conversion11/1 -> Rate Transition12/1  "tau_engine_target"
  tau_brake/1 -> Memory8/1
  Data Type Conversion6/1 -> Rate Transition7/1  "trans_shifer_position"
  w_gearbox_output_radps/1 -> Memory1/1
  Constant/1 -> Manual Switch1/2
  t_engine_water_k/1 -> Memory4/1
  Data Type Conversion10/1 -> Rate Transition11/1  "w_engine_idle_radps"
  w_engine_radps/1 -> Memory9/1
  tau_engine_max_pos/1 -> Memory14/1
  Model/12 -> Data Type Conversion28/1
  Model/7 -> Data Type Conversion23/1
  Model/8 -> Data Type Conversion24/1
  Data Type Conversion12/1 -> Rate Transition13/1  "tau_engine"
  Data Type Conversion3/1 -> Rate Transition4/1  "t_trans_fluid_k"
  Data Type Conversion4/1 -> Rate Transition5/1  "t_engine_water_k"
  Data Type Conversion7/1 -> Rate Transition8/1, mps2rps/1  "v_vehicle_mps"
  Mux/1 -> tq_clutch_cap/1  "tq_clutch_cap"
  Data Type Conversion19/1 -> p_line/1  "p_line"
  Data Type Conversion20/1 -> i_actuator/1  "i_actuator"
  Data Type Conversion21/1 -> i_eop/1  "i_eop"
  Data Type Conversion22/1 -> q_cooler_trans_fluid/1  "q_cooler_trans_fluid"
  Data Type Conversion23/1 -> q_cooler_engine_water/1  "q_cooler_engine_water"
  Data Type Conversion24/1 -> tq_engine_max_req/1  "tq_engine_max_req"
  Data Type Conversion25/1 -> tq_engine_min_req/1  "tq_engine_min_req"
  Data Type Conversion26/1 -> r_engine_target/1  "r_engine_target"
  Data Type Conversion27/1 -> tq_trans_input/1  "tq_trans_input"
  Data Type Conversion28/1 -> [tScope_AT_GearRatio], gear_ratio/1  "gear_ratio"
  Memory/1 -> Data Type Conversion1/1
  Memory1/1 -> Data Type Conversion2/1
  Memory2/1 -> Data Type Conversion15/1
  Memory3/1 -> Data Type Conversion3/1
  Memory4/1 -> Data Type Conversion4/1
  Memory5/1 -> Data Type Conversion5/1
  Memory6/1 -> Data Type Conversion6/1
  Memory7/1 -> Data Type Conversion7/1
  Memory8/1 -> Data Type Conversion8/1
  Memory9/1 -> Data Type Conversion9/1
  Memory10/1 -> Data Type Conversion10/1
  Memory11/1 -> Data Type Conversion11/1
  Memory12/1 -> Data Type Conversion12/1
  Memory13/1 -> Data Type Conversion13/1
  Memory14/1 -> Data Type Conversion14/1
  Data Type Conversion18/1 -> f_synchro_n/1  "f_synchro_n"
  Data Type Conversion17/1 -> Demux/1  "tq_clutch_cap"
  Demux/11 -> lock_up_cap/1  "lock_up_cap"
  Demux/1 -> Mux/1
  Demux/2 -> Mux/2
  Demux/3 -> Mux/3
  Demux/4 -> Mux/4
  Demux/5 -> Mux/5
  Demux/6 -> Mux/6
  Demux/7 -> Mux/7
  Demux/8 -> Mux/8
  Demux/9 -> Mux/9
  Demux/10 -> Mux/10
  Rate Transition/1 -> Model/1
  Rate Transition1/1 -> Model/2
  Rate Transition2/1 -> Model/3
  Rate Transition3/1 -> Model/4
  Rate Transition4/1 -> Model/5
  Rate Transition5/1 -> Model/6
  Rate Transition6/1 -> Model/7
  Rate Transition7/1 -> Model/8
  Rate Transition8/1 -> Model/9
  Rate Transition9/1 -> Model/10
  Rate Transition10/1 -> Model/11
  Rate Transition11/1 -> Model/12
  Rate Transition12/1 -> Model/13
  Rate Transition13/1 -> Model/14
  Rate Transition14/1 -> Model/15
  Rate Transition15/1 -> Model/16
  Data Type Conversion29/1 -> flag_lock_up/1  "flag_lock_up"

== system TRAMI_STEP_AT_vehicle_ver01_Jmaab_R2018b/Vehicle/ENG_PNT/ENG_Plant/Cal_FuelComsunption ==
  w_ENG_PNT_radps : Inport
  trq_ENG : Inport  Port=2
  flag_fuelcut : Inport  Port=3
  flag_IdleStop : Inport  Port=4
  timing_ignition : Inport  Port=5
  1-D Lookup Table1 : Lookup_n-D  NumberOfTableDimensions=1  BreakpointsForDimension1=ENG_PNT_trq_fluc_Nm_table_x_spk_tim  Table=ENG_PNT_trq_fluc_Nm_table  RndMeth=Simplest  InputSameDT=on
  Map_FuelRate : Lookup_n-D  BreakpointsForDimension1=ENG_PNT_FuelCon_gps_map_y_trq_Nm  BreakpointsForDimension2=ENG_PNT_FuelCon_gps_map_x_pri_rpm  Table=ENG_PNT_FuelCon_gps_map  RndMeth=Simplest  InputSameDT=on
  Not_cal1 : Subsystem
  Not_cal2 : Subsystem
  Product : Product  Inputs=3  RndMeth=Zero
  Product1 : Product  Inputs=*/  RndMeth=Zero
  radpsec2rpm : Gain  Gain=radpsec2rpm
  FuelComsunption : Outport
  wires:
  trq_ENG/1 -> Product1/1
  radpsec2rpm/1 -> Map_FuelRate/2
  w_ENG_PNT_radps/1 -> radpsec2rpm/1
  Product/1 -> FuelComsunption/1
  Not_cal2/1(Out1) -> Product/3
  Not_cal1/1(Out1) -> Product/2
  flag_fuelcut/1 -> Not_cal1/1(In1)
  flag_IdleStop/1 -> Not_cal2/1(In1)
  timing_ignition/1 -> 1-D Lookup Table1/1
  1-D Lookup Table1/1 -> Product1/2
  Product1/1 -> Map_FuelRate/1
  Map_FuelRate/1 -> Product/1

== system TRAMI_STEP_AT_vehicle_ver01_Jmaab_R2018b/Vehicle/ENG_PNT/ENG_Plant/Cal_trq_ENG_jiku ==
  note: エンジン軸トルクマップ
  open_throttle_per : Inport
  flag_fuelcut : Inport  Port=2
  flag_IdleStop : Inport  Port=3
  timing_ignition : Inport  Port=4
  w_ENG_PNT_radps : Inport  Port=5
  1-D Lookup Table : Lookup_n-D  NumberOfTableDimensions=1  BreakpointsForDimension1=ENG_PNT_trq_fluc_Nm_table_x_spk_tim  Table=ENG_PNT_trq_fluc_Nm_table  RndMeth=Simplest  InputSameDT=on
  2-D Lookup Table : Lookup_n-D  BreakpointsForDimension1=ENG_PNT_trq_Nm_map_y_throttle  BreakpointsForDimension2=ENG_PNT_trq_Nm_map_x_rpm  Table=ENG_PNT_trq_Nm_map  ExtrapMethod=Clip  UseLastTableValue=on  RndMeth=Simplest  InputSameDT=on
  Model Info : simulink/Model-Wide Utilities/Model Info  Frame=on  DisplayStringWithTags=|  HorizontalTextAlignment=Left  LeftAlignmentValue=0.02
      | 【注記】
      | ・燃料カット時はスロットル開度を0としてエンジンフリクションを付加
      | ・点火タイミングによるトルク変動を想定
      | ・エンジン軸トルクマップの使用
  Not_cal : Subsystem
  Not_cal1 : Subsystem
  Product : Product  RndMeth=Zero
  Product1 : Product  RndMeth=Zero
  Product2 : Product  RndMeth=Zero
  Saturation : Saturate  UpperLimit=ENG_CNT_Throttle_UL  LowerLimit=ENG_CNT_Throttle_LL
  radpsec2rpm : Gain  Gain=radpsec2rpm
  trq_ENG_PNT_Nm : Outport
  wires:
  w_ENG_PNT_radps/1 -> radpsec2rpm/1
  2-D Lookup Table/1 -> Product1/1
  open_throttle_per/1 -> Product/1
  Saturation/1 -> 2-D Lookup Table/1
  radpsec2rpm/1 -> 2-D Lookup Table/2
  timing_ignition/1 -> 1-D Lookup Table/1
  1-D Lookup Table/1 -> Product1/2
  Product/1 -> Saturation/1
  Product2/1 -> Product/2
  flag_fuelcut/1 -> Not_cal/1(In1)
  Not_cal/1(Out1) -> Product2/1
  flag_IdleStop/1 -> Not_cal1/1(In1)
  Not_cal1/1(Out1) -> Product2/2
  Product1/1 -> trq_ENG_PNT_Nm/1  "trq_ENG_PNT_Nm"

== system TRAMI_STEP_AT_vehicle_ver01_Jmaab_R2018b/Driver/Caliculate_Opeining_Accel/FF/Cal_M_ENG_jiku2/Subsystem ==
  In1 : Inport
  Constant1 : Constant  Value=0
  Switch : Switch  Criteria=u2 > Threshold  Threshold=0.1
  Out1 : Outport
  wires:
  Switch/1 -> Out1/1
  Constant1/1 -> Switch/3
  In1/1 -> Switch/2, Switch/1

== system TRAMI_STEP_AT_vehicle_ver01_Jmaab_R2018b/Vehicle/ALT_PNT/Subsystem/I_alt_cal/Cal_I_alt_P_control ==
  note: 目標電圧よりもオルタネータ電圧が低い場合電流をPI制御で出力
      | 高い場合は、電流を0とする
  V_delt_tgt : Inport
  Gain : Gain  Gain=ALT_PNT_Gain_Alt_v_del
  Transfer Fcn : TransferFcn  Denominator=[ALT_PNT_Tau_Alternator_V_tgt_s 1]
  I_alt_base : Outport
  wires:
  Gain/1 -> I_alt_base/1
  V_delt_tgt/1 -> Transfer Fcn/1
  Transfer Fcn/1 -> Gain/1

== system TRAMI_STEP_AT_vehicle_ver01_Jmaab_R2018b/Vehicle/ALT_PNT/Subsystem/I_alt_cal/Cal_I_alt_base ==
  note: 目標電圧よりもオルタネータ電圧が低い場合電流をPI制御で出力
      | 高い場合は、電流を0とする
  V_delt_tgt : Inport
  Constant : Constant  Value=0
  Gain : Gain  Gain=1/BT_PNT_Lo_R_lo_batt_ohm
  MinMax : MinMax  Function=max  Inputs=2
  Switch : Switch  Criteria=u2 > Threshold
  Transfer Fcn : TransferFcn  Denominator=[ALT_PNT_Tau_Alternator_V_tgt_s 1]
  I_alt_base : Outport
  wires:
  MinMax/1 -> I_alt_base/1
  Gain/1 -> Switch/1
  V_delt_tgt/1 -> Transfer Fcn/1
  Constant/1 -> MinMax/2, Switch/3
  Switch/1 -> MinMax/1
  Transfer Fcn/1 -> Switch/2, Gain/1

== system TRAMI_STEP_AT_vehicle_ver01_Jmaab_R2018b/Vehicle/CNT/ENG_CNT/ENG_Cntrl/Caliculate_Idle_Speed ==
  note: 目標アイドル回転数
  note: ○目標回転数に対するP制御
  note: 補機負荷やNDの時の負荷によるアイドル安定化処理を入れる
      | パワーデマンドで締結
  per_throttle_base : Inport
  n_eng_rpm : Inport  Port=2
  flag_Lockup : Inport  Port=3
  flag_IdleStop : Inport  Port=4
  IdleSpeed : Constant  Value=ENG_CNT_IdleSpeed_Const
  Subsystem : Subsystem
  Subsystem1 : Subsystem
  Subtract : Sum  Inputs=+-
  per_isc_[%] : Outport
  IdleSpeed_Target : Outport  Port=2
  wires:
  IdleSpeed/1 -> IdleSpeed_Target/1, Subsystem1/1(omg_tgt_idle), Subtract/1  "IdleSpeed_Target"
  n_eng_rpm/1 -> Subsystem1/2(n_eng_rpm), Subtract/2
  Subtract/1 -> Subsystem/1(del_omg_engine)
  per_throttle_base/1 -> Subsystem1/3(per_throttle_base)
  flag_Lockup/1 -> Subsystem1/4(flag_Lockup)
  Subsystem1/1(flag_idle_fb) -> Subsystem/2(flag_idle_fb)
  flag_IdleStop/1 -> Subsystem1/5(flag_IdleStop)
  Subsystem/1(per_isc_[%]) -> per_isc_[%]/1

== system TRAMI_STEP_AT_vehicle_ver01_Jmaab_R2018b/Vehicle/CNT/ENG_CNT/ENG_Cntrl/Set_Fuel_Cut ==
  note: ○減速時のフューエルカット条件
      | 　・停車中でない
      | 　・回転数がある回転数以上
      | 　・アクセル開度がOFF
  v_vehicle : Inport
  n_eng_rpm : Inport  Port=2
  per_throttle_base : Inport  Port=3
  Constant1 : Constant  Value=ENG_CNT_V_vhicle_fuelcut_kmph
  Constant4 : Constant  Value=ENG_CNT_omg_eng_fuelcut_rpm
  Constant6 : Constant  Value=ENG_CNT_per_throttle_fuelcut
  Logical Operator : Logic  Inputs=3  AllPortsSameDT=off  OutDataTypeStr=boolean
  Relational Operator1 : RelationalOperator  Operator=<=  OutDataTypeStr=boolean  RndMeth=Nearest
  Relational Operator2 : RelationalOperator  OutDataTypeStr=boolean  RndMeth=Nearest
  Relational Operator3 : RelationalOperator  OutDataTypeStr=boolean  RndMeth=Nearest
  flag_fuelcut : Outport
  wires:
  n_eng_rpm/1 -> Relational Operator2/1
  per_throttle_base/1 -> Relational Operator1/1
  Constant6/1 -> Relational Operator1/2
  Relational Operator1/1 -> Logical Operator/3
  Relational Operator2/1 -> Logical Operator/2
  Logical Operator/1 -> flag_fuelcut/1
  Constant1/1 -> Relational Operator3/2
  v_vehicle/1 -> Relational Operator3/1
  Relational Operator3/1 -> Logical Operator/1
  Constant4/1 -> Relational Operator2/2

== system TRAMI_STEP_AT_vehicle_ver01_Jmaab_R2018b/Vehicle/CNT/ENG_CNT/ENG_Cntrl/Set_Idle_Stop ==
  note: ○アイドリングストップ制御
      | 　停車時＋ブレーキを踏んでいるとき、アイドリングストップ
  v_vehicle : Inport
  per_brake : Inport  Port=2
  Constant : Constant  Value=ENG_CNT_V_car_idlestop_kmph
  Constant1 : Constant  Value=ENG_CNT_brak_idlestop
  Constant2 : Constant  Value=ENG_CNT_flag_idle_stop_exe
  Logical Operator : Logic  Inputs=3  AllPortsSameDT=off  OutDataTypeStr=boolean
  Relational Operator : RelationalOperator  Operator=<  OutDataTypeStr=boolean  RndMeth=Nearest
  Relational Operator1 : RelationalOperator  OutDataTypeStr=boolean  RndMeth=Nearest
  flag_IdleStop : Outport
  wires:
  Relational Operator/1 -> Logical Operator/2
  Logical Operator/1 -> flag_IdleStop/1
  v_vehicle/1 -> Relational Operator/1
  per_brake/1 -> Relational Operator1/1
  Constant/1 -> Relational Operator/2
  Constant1/1 -> Relational Operator1/2
  Relational Operator1/1 -> Logical Operator/3
  Constant2/1 -> Logical Operator/1

== system TRAMI_STEP_AT_vehicle_ver01_Jmaab_R2018b/Vehicle/CNT/ENG_CNT/ENG_Cntrl/Starter ==
  note: サンプリング時間
  note: 時間リセット
  note: アイドリングフラグがON→OFFに
      | 切り替わり時スターターON開始
  note: スタータ開始時間
  note: スタータ開始時間から
      | ある時間超えたらOFF
  note: アイドリングフラグがON→OFFに切り替わり時スターターON開始.ある時間を超えたらOFF
  flag_idlestop : Inport
  n_eng_rpm : Inport  Port=2
  Constant2 : Constant  Value=ENG_CNT_Starter_timer_Const_s
  Constant4 : Constant  Value=sampling_time
  Constant5 : Constant  Value=0
  Constant6 : Constant  Value=OFF
  Constant7 : Constant  Value=ON
  IdleSpeed : Constant  Value=ENG_CNT_IdleSpeed_Const/2
  Logical Operator : Logic  Inputs=3  AllPortsSameDT=off  OutDataTypeStr=boolean
  Logical Operator1 : Logic  Operator=NOT  AllPortsSameDT=off  OutDataTypeStr=boolean
  Memory : Memory  InitialCondition=1000
  Memory1 : Memory  InheritSampleTime=on
  Relational Operator1 : RelationalOperator  Operator=<=  OutDataTypeStr=boolean  RndMeth=Nearest
  Relational Operator2 : RelationalOperator  Operator=<  OutDataTypeStr=boolean  RndMeth=Nearest
  Sum5 : Sum  Inputs=|++
  Switch3 : Switch  Criteria=u2 > Threshold  Threshold=0.5
  Switch4 : Switch  Criteria=u2 > Threshold  Threshold=0.5
  flag_ON_Starter : Outport
  wires:
  Switch4/1 -> flag_ON_Starter/1
  Memory/1 -> Sum5/2
  Constant4/1 -> Sum5/1
  Constant5/1 -> Switch3/1
  Sum5/1 -> Switch3/3
  Switch3/1 -> Relational Operator1/1, Memory/1
  Memory1/1 -> Logical Operator/2
  Logical Operator1/1 -> Logical Operator/1
  flag_idlestop/1 -> Memory1/1, Logical Operator1/1
  Logical Operator/1 -> Switch3/2
  Constant2/1 -> Relational Operator1/2
  Relational Operator1/1 -> Switch4/2
  Constant7/1 -> Switch4/1
  Constant6/1 -> Switch4/3
  n_eng_rpm/1 -> Relational Operator2/1
  IdleSpeed/1 -> Relational Operator2/2
  Relational Operator2/1 -> Logical Operator/3

== system TRAMI_STEP_AT_vehicle_ver01_Jmaab_R2018b/Vehicle/ENG_PNT/ENG_Plant/Cal_FuelComsunption/Not_cal1 ==
  In1 : Inport
  Constant : Constant  Value=0
  Constant1 : Constant
  Switch : Switch  Criteria=u2 > Threshold  Threshold=0.5
  Out1 : Outport
  wires:
  Constant1/1 -> Switch/3
  Constant/1 -> Switch/1
  Switch/1 -> Out1/1
  In1/1 -> Switch/2

== system TRAMI_STEP_AT_vehicle_ver01_Jmaab_R2018b/Vehicle/ENG_PNT/ENG_Plant/Cal_FuelComsunption/Not_cal2 ==
  In1 : Inport
  Constant : Constant  Value=0
  Constant1 : Constant
  Switch : Switch  Criteria=u2 > Threshold  Threshold=0.5
  Out1 : Outport
  wires:
  In1/1 -> Switch/2
  Switch/1 -> Out1/1
  Constant/1 -> Switch/1
  Constant1/1 -> Switch/3

== system TRAMI_STEP_AT_vehicle_ver01_Jmaab_R2018b/Vehicle/ENG_PNT/ENG_Plant/Cal_trq_ENG_jiku/Not_cal ==
  In1 : Inport
  Constant : Constant  Value=0
  Constant1 : Constant
  Switch : Switch  Criteria=u2 > Threshold  Threshold=0.5
  Out1 : Outport
  wires:
  In1/1 -> Switch/2
  Switch/1 -> Out1/1
  Constant/1 -> Switch/1
  Constant1/1 -> Switch/3
